simulink model "EX_6_3"  (R2013a)
settings: Solver=ode45  StartTime=0.0  StopTime=3  RelTol=1e-3
settings Model: Creator=Reza  LastModifiedBy=Reza

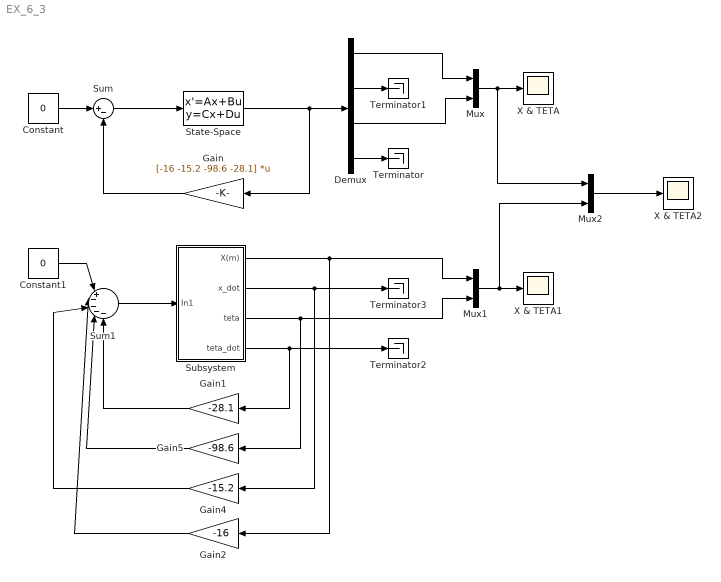
== system EX_6_3 ==
  Constant : Constant  Value=0
  Constant1 : Constant  Value=0
  Demux : Demux
  Gain : Gain  Gain=[-16 -15.2 -98.6 -28.1]  Multiplication=Matrix(K*u)
  Gain1 : Gain  Gain=-28.1
  Gain2 : Gain  Gain=-16
  Gain4 : Gain  Gain=-15.2
  Gain5 : Gain  Gain=-98.6
  Mux : Mux  Inputs=2
  Mux1 : Mux  Inputs=2
  Mux2 : Mux  Inputs=2
  State-Space : StateSpace  A=[0 1 0 0;0 0 -9.8 0;0 0 0 1;0 0 19.6 0]  B=[0;1;0;-1]  C=[1 0 0 0;0 1 0 0;0 0 1 0;0 0 0 1]  D=[0;0;0;0]  X0=[0 0 0.26 0]
  Subsystem : Subsystem
  Sum : Sum  Inputs=|+-
  Sum1 : Sum  Inputs=|+----
  Terminator{,1..3} (4 alike) : Terminator
  X & TETA : Scope
      settings: TimeRange=3  YMin=-0.2  YMax=0.6000000000000001
  X & TETA1 : Scope
      settings: YMin=0  YMax=7e+10
  X & TETA2 : Scope
      settings: SaveName=ScopeData2
  wires:
  Constant/1 -> Sum/1
  Sum/1 -> State-Space/1
  Demux/2 -> Terminator1/1
  Demux/4 -> Terminator/1
  Demux/1 -> Mux/1
  Demux/3 -> Mux/2
  Mux/1 -> Mux2/1, X & TETA/1
  Sum1/1 -> Subsystem/1(In1)
  Mux1/1 -> Mux2/2, X & TETA1/1
  Constant1/1 -> Sum1/1
  Mux2/1 -> X & TETA2/1
  Gain/1 -> Sum/2
  State-Space/1 -> Gain/1, Demux/1
  Gain1/1 -> Sum1/5
  Gain5/1 -> Sum1/4
  Gain4/1 -> Sum1/3
  Gain2/1 -> Sum1/2
  Subsystem/1(X(m)) -> Gain2/1, Mux1/1
  Subsystem/3(teta) -> Gain5/1, Mux1/2
  Subsystem/2(x_dot) -> Gain4/1, Terminator3/1
  Subsystem/4(teta_dot) -> Gain1/1, Terminator2/1

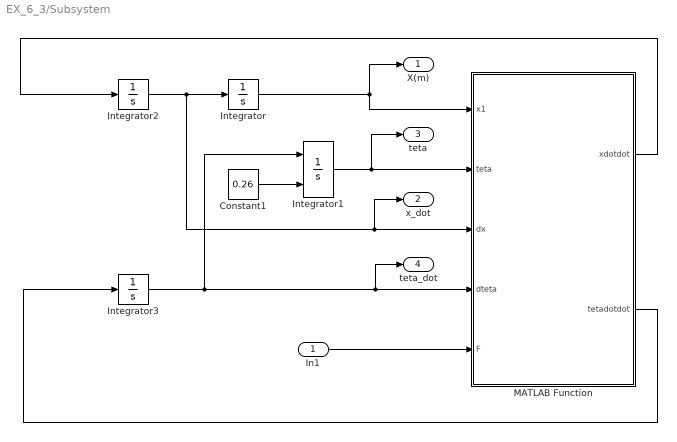
== system EX_6_3/Subsystem ==
  In1 : Inport
  Constant1 : Constant  Value=0.26
  Integrator : Integrator
  Integrator1 : Integrator  InitialConditionSource=external  InitialCondition=0.1
  Integrator2 : Integrator
  Integrator3 : Integrator
  MATLAB Function : MATLAB Function  TreatAsAtomicUnit=on
  X(m) : Outport
  x_dot : Outport  Port=2
  teta : Outport  Port=3
  teta_dot : Outport  Port=4
  wires:
  Integrator3/1 -> teta_dot/1, MATLAB Function/4(dteta), Integrator1/1
  Constant1/1 -> Integrator1/2
  Integrator1/1 -> teta/1, MATLAB Function/2(teta)
  In1/1 -> MATLAB Function/5(F)
  Integrator/1 -> X(m)/1, MATLAB Function/1(x1)
  Integrator2/1 -> Integrator/1, x_dot/1, MATLAB Function/3(dx)
  MATLAB Function/1(xdotdot) -> Integrator2/1
  MATLAB Function/2(tetadotdot) -> Integrator3/1

== matlab function EX_6_3/Subsystem/MATLAB Function ==
  data: x1 input; xdotdot output; tetadotdot output; teta input; dx input; dteta input; F input
function [xdotdot,tetadotdot] = fcn(x1,teta,dx,dteta,F)
%#codegen
xdot = dx;
tetadot = dteta;
xdotdot = (F+sin(teta)*((dteta)^2)-9.8*sin(teta)*cos(teta))/(2-(cos(teta))^2);
tetadotdot = (-F*cos(teta)-sin(teta)*cos(teta)*((dteta)^2)+19.6*sin(teta))/(2-(cos(teta))^2);
